simulink model "assignment_1"  (R2022a)
settings: Solver=FixedStepAuto  StartTime=0.0  StopTime=inf  FixedStep=1e-3  RelTol=1e-3  EnableMultiTasking=on
undefined symbols (not defined in the file): D0, D1, D10, D11, D12, D13, D2, D3, D4, D5, D6, D7, D8, D9, PTA0, PTA1, PTA2, PTB23, PTB9, PTC16, PTC17, PTC2, PTC3, PTC4, PTD0, PTD1, PTD2, PTD3
libraries: frdmk64flib x16
settings Model: ExtModeTrigDuration=5  Creator=Xu Yue  LastModifiedBy=Xu Yue
settings OptimizationCC: EnhancedBackFolding=on  PassReuseOutputArgsAs=Individual arguments  ZeroExternalMemoryAtStartup=off  ZeroInternalMemoryAtStartup=off  MaxStackSize=64  OptimizeBlockOrder=speed  DifferentSizesBufferReuse=on  OptimizationCustomize=off  EfficientTunableParamExpr=on
settings DebuggingCC: ParameterTunabilityLossMsg=error
settings HardwareCC: ProdBitPerPointer=32  ProdBitPerSizeT=32  ProdBitPerPtrDiffT=32  ProdLargestAtomicInteger=Long  ProdLargestAtomicFloat=Double  ProdWordSize=32  ProdHWDeviceType=ARM Compatible->ARM Cortex
settings SFSimCC: MATLABDynamicMemAlloc=off
settings RTWCC: SystemTargetFile=ert.tlc  HardwareBoard=NXP FRDM-K64F  TLCOptions="-aInlineSetEventsForThisBaseRateFcn=TLC_FALSE -aSuppressMultiTaskScheduler=TLC_FALSE  -aRateBasedStepFcn=0"  TemplateMakefile=ert_default_tmf  Toolchain=GNU Tools for ARM Embedded Processors
settings CodeAppCC: ForceParamTrailComments=on  IgnoreCustomStorageClasses=off  OperatorAnnotations=on  SimulinkDataObjDesc=on  SFDataObjDesc=on  InsertBlockDesc=on
settings ERTTargetCC: SupportContinuousTime=on  ExtModeTransport=4  ExtModeMexFile=sendToCommService

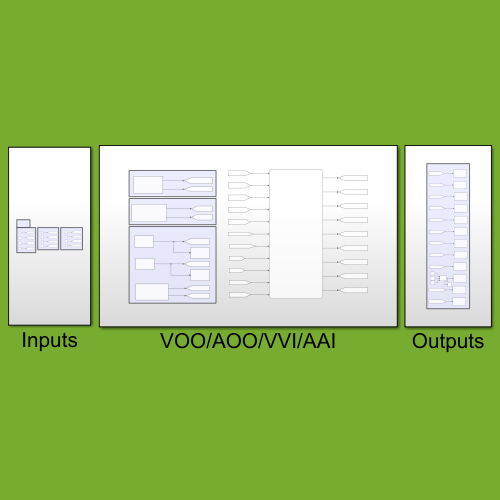
[thumbnail: Simulink's stored preview of the top-level diagram]
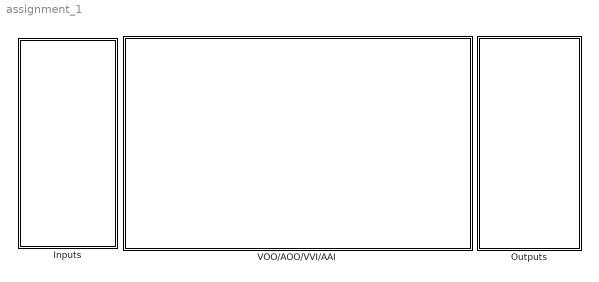
== system assignment_1 ==
  Inputs : Subsystem
  Outputs : Subsystem
  VOO/AOO/VVI/AAI : Subsystem

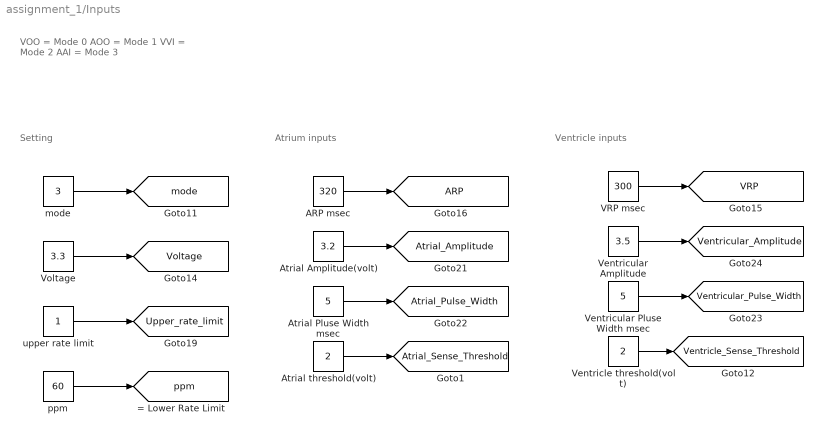
== system assignment_1/Inputs ==
  note: VOO = Mode 0
      | AOO = Mode 1
      | VVI = Mode 2
      | AAI = Mode 3
  note: Atrium inputs
  note: Setting
  note: Ventricle inputs
  ARP msec : Constant  Value=320
  Atrial Amplitude(volt) : Constant  Value=3.2
  Atrial Pluse Width msec : Constant  Value=5
  Atrial threshold(volt) : Constant  Value=2
  VRP msec : Constant  Value=300
  Ventricle threshold(volt) : Constant  Value=2
  Ventricular Amplitude : Constant  Value=3.5
  Ventricular Pluse Width msec : Constant  Value=5
  Voltage : Constant  Value=3.3
  mode : Constant  Value=3
  ppm : Constant  Value=60
  upper rate limit : Constant
  tag scope: ARP=global, Atrial_Amplitude=global, Atrial_Pulse_Width=global, Atrial_Sense_Threshold=global, Upper_rate_limit=global, VRP=global, Ventricle_Sense_Threshold=global, Ventricular_Amplitude=global, Ventricular_Pulse_Width=global, Voltage=global, mode=global, ppm=global
  wires:
  Ventricular Pluse Width msec/1 -> [Ventricular_Pulse_Width]
  Voltage/1 -> [Voltage]
  ppm/1 -> [ppm]
  mode/1 -> [mode]
  Ventricular Amplitude/1 -> [Ventricular_Amplitude]
  VRP msec/1 -> [VRP]
  upper rate limit/1 -> [Upper_rate_limit]
  Atrial Pluse Width msec/1 -> [Atrial_Pulse_Width]
  ARP msec/1 -> [ARP]
  Atrial Amplitude(volt)/1 -> [Atrial_Amplitude]
  Atrial threshold(volt)/1 -> [Atrial_Sense_Threshold]
  Ventricle threshold(volt)/1 -> [Ventricle_Sense_Threshold]

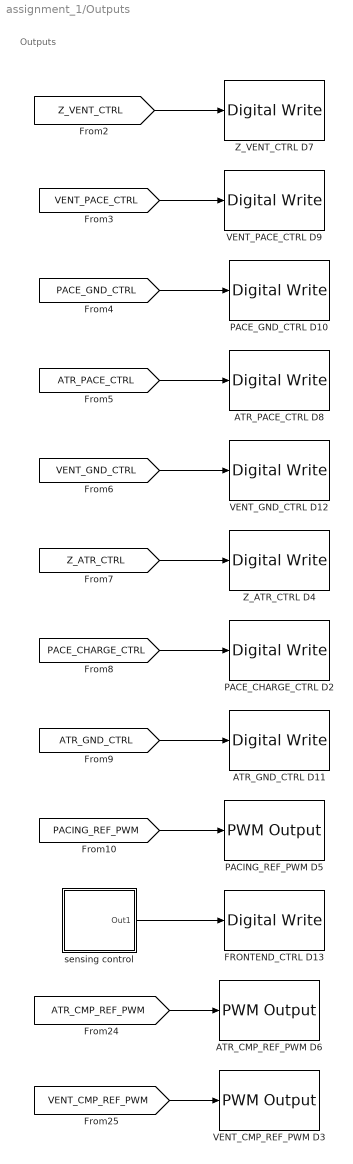
== system assignment_1/Outputs ==
  note: Outputs
  ATR_CMP_REF_PWM D6 : frdmk64flib/PWM Output  Whichpin=PTC2 (D6)  InitialFrequency=2000  InitialDutyCycle=0
  ATR_GND_CTRL D11 : frdmk64flib/Digital Write  Whichpin=PTD2 (D11)
  ATR_PACE_CTRL D8 : frdmk64flib/Digital Write  Whichpin=PTA0 (D8)
  FRONTEND_CTRL D13 : frdmk64flib/Digital Write  Whichpin=PTD1 (D13)
  PACE_CHARGE_CTRL D2 : frdmk64flib/Digital Write  Whichpin=PTB9 (D2)
  PACE_GND_CTRL D10 : frdmk64flib/Digital Write  Whichpin=PTD0 (D10)
  PACING_REF_PWM D5 : frdmk64flib/PWM Output  Whichpin=PTA2 (D5)  InitialFrequency=2000  InitialDutyCycle=0
  VENT_CMP_REF_PWM D3 : frdmk64flib/PWM Output  Whichpin=PTA1 (D3)  InitialFrequency=2000  InitialDutyCycle=0
  VENT_GND_CTRL D12 : frdmk64flib/Digital Write  Whichpin=PTD3 (D12)
  "VENT_PACE_CTRL D9  " : frdmk64flib/Digital Write  Whichpin=PTC4 (D9)
  Z_ATR_CTRL D4 : frdmk64flib/Digital Write  Whichpin=PTB23 (D4)
  Z_VENT_CTRL D7 : frdmk64flib/Digital Write  Whichpin=PTC3 (D7)
  sensing control : Subsystem
  wires:
  [VENT_GND_CTRL] -> VENT_GND_CTRL D12/1
  [ATR_PACE_CTRL] -> ATR_PACE_CTRL D8/1
  [PACE_CHARGE_CTRL] -> PACE_CHARGE_CTRL D2/1
  [VENT_PACE_CTRL] -> "VENT_PACE_CTRL D9  "/1
  [Z_VENT_CTRL] -> Z_VENT_CTRL D7/1
  [PACE_GND_CTRL] -> PACE_GND_CTRL D10/1
  [Z_ATR_CTRL] -> Z_ATR_CTRL D4/1
  [PACING_REF_PWM] -> PACING_REF_PWM D5/1
  [ATR_CMP_REF_PWM] -> ATR_CMP_REF_PWM D6/1
  [VENT_CMP_REF_PWM] -> VENT_CMP_REF_PWM D3/1
  [ATR_GND_CTRL] -> ATR_GND_CTRL D11/1
  sensing control/1(Out1) -> FRONTEND_CTRL D13/1

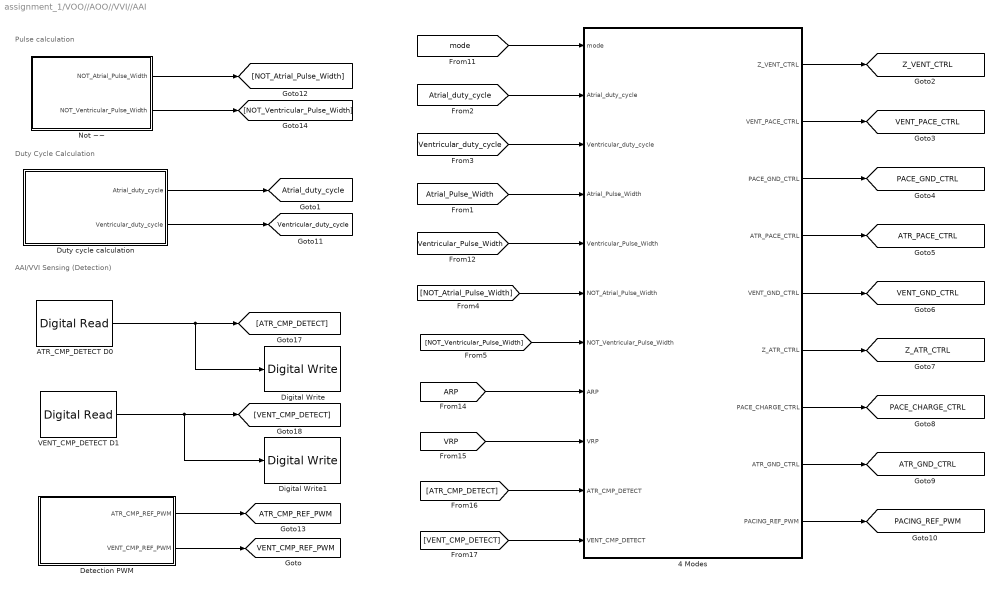
== system assignment_1/VOO//AOO//VVI//AAI ==
  note: Duty Cycle Calculation
  note: Pulse calculation
  note: AAI/VVI Sensing (Detection)
  4 Modes : Stateflow chart  TreatAsAtomicUnit=on
  ATR_CMP_DETECT D0 : frdmk64flib/Digital Read  Whichpin=PTC16 (D0)  SampleTime=-1
  Detection PWM : Subsystem
  Digital Write : frdmk64flib/Digital Write  Whichpin=RED_LED
  Digital Write1 : frdmk64flib/Digital Write  Whichpin=BLUE_LED
  Duty cycle calculation : Subsystem
  Not ~~ : Subsystem
  VENT_CMP_DETECT D1 : frdmk64flib/Digital Read  Whichpin=PTC17 (D1)  SampleTime=-1
  tag scope: ATR_CMP_REF_PWM=global, ATR_GND_CTRL=global, ATR_PACE_CTRL=global, Atrial_duty_cycle=global, PACE_CHARGE_CTRL=global, PACE_GND_CTRL=global, PACING_REF_PWM=global, VENT_CMP_REF_PWM=global, VENT_GND_CTRL=global, VENT_PACE_CTRL=global, Ventricular_duty_cycle=global, Z_ATR_CTRL=global, Z_VENT_CTRL=global
  wires:
  4 Modes/5(VENT_GND_CTRL) -> [VENT_GND_CTRL]
  4 Modes/1(Z_VENT_CTRL) -> [Z_VENT_CTRL]
  4 Modes/8(ATR_GND_CTRL) -> [ATR_GND_CTRL]
  Detection PWM/1(ATR_CMP_REF_PWM) -> [ATR_CMP_REF_PWM]
  [mode] -> 4 Modes/1(mode)
  4 Modes/6(Z_ATR_CTRL) -> [Z_ATR_CTRL]
  4 Modes/3(PACE_GND_CTRL) -> [PACE_GND_CTRL]
  4 Modes/9(PACING_REF_PWM) -> [PACING_REF_PWM]
  [ATR_CMP_DETECT] -> 4 Modes/10(ATR_CMP_DETECT)
  4 Modes/2(VENT_PACE_CTRL) -> [VENT_PACE_CTRL]
  ATR_CMP_DETECT D0/1 -> Digital Write/1, [ATR_CMP_DETECT]
  [VENT_CMP_DETECT] -> 4 Modes/11(VENT_CMP_DETECT)
  [Atrial_Pulse_Width] -> 4 Modes/4(Atrial_Pulse_Width)
  [ARP] -> 4 Modes/8(ARP)
  [Ventricular_Pulse_Width] -> 4 Modes/5(Ventricular_Pulse_Width)
  4 Modes/4(ATR_PACE_CTRL) -> [ATR_PACE_CTRL]
  [VRP] -> 4 Modes/9(VRP)
  4 Modes/7(PACE_CHARGE_CTRL) -> [PACE_CHARGE_CTRL]
  Detection PWM/2(VENT_CMP_REF_PWM) -> [VENT_CMP_REF_PWM]
  Duty cycle calculation/1(Atrial_duty_cycle) -> [Atrial_duty_cycle]
  Duty cycle calculation/2(Ventricular_duty_cycle) -> [Ventricular_duty_cycle]
  [Atrial_duty_cycle] -> 4 Modes/2(Atrial_duty_cycle)
  [Ventricular_duty_cycle] -> 4 Modes/3(Ventricular_duty_cycle)
  Not ~~/1(NOT_Atrial_Pulse_Width) -> [NOT_Atrial_Pulse_Width]
  Not ~~/2(NOT_Ventricular_Pulse_Width) -> [NOT_Ventricular_Pulse_Width]
  [NOT_Atrial_Pulse_Width] -> 4 Modes/6(NOT_Atrial_Pulse_Width)
  [NOT_Ventricular_Pulse_Width] -> 4 Modes/7(NOT_Ventricular_Pulse_Width)
  VENT_CMP_DETECT D1/1 -> Digital Write1/1, [VENT_CMP_DETECT]

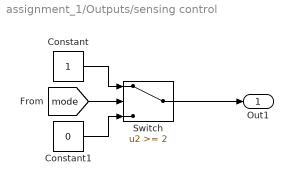
== system assignment_1/Outputs/sensing control ==
  Constant : Constant
  Constant1 : Constant  Value=0
  Switch : Switch  Threshold=2  SaturateOnIntegerOverflow=off  InputSameDT=off
  Out1 : Outport
  wires:
  Constant/1 -> Switch/1
  Constant1/1 -> Switch/3
  [mode] -> Switch/2
  Switch/1 -> Out1/1

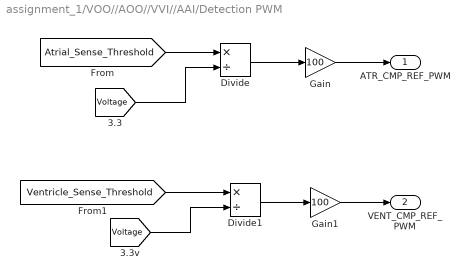
== system assignment_1/VOO//AOO//VVI//AAI/Detection PWM ==
  Divide : Product  Inputs=*/  RndMeth=Zero  SaturateOnIntegerOverflow=on
  Divide1 : Product  Inputs=*/  RndMeth=Zero  SaturateOnIntegerOverflow=on
  Gain : Gain  Gain=100
  Gain1 : Gain  Gain=100
  ATR_CMP_REF_PWM : Outport
  VENT_CMP_REF_PWM : Outport  Port=2
  wires:
  Divide/1 -> Gain/1
  Gain/1 -> ATR_CMP_REF_PWM/1
  [Voltage] -> Divide1/2
  Divide1/1 -> Gain1/1
  Gain1/1 -> VENT_CMP_REF_PWM/1
  [Voltage] -> Divide/2
  [Atrial_Sense_Threshold] -> Divide/1
  [Ventricle_Sense_Threshold] -> Divide1/1

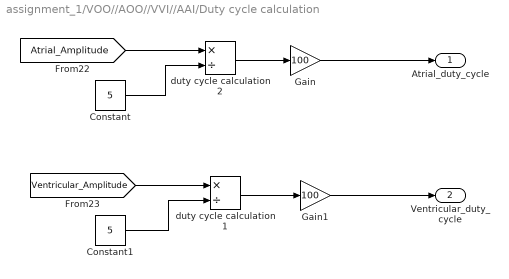
== system assignment_1/VOO//AOO//VVI//AAI/Duty cycle calculation ==
  Constant : Constant  Value=5
  Constant1 : Constant  Value=5
  Gain : Gain  Gain=100
  Gain1 : Gain  Gain=100
  duty cycle calculation1 : Product  Inputs=*/  RndMeth=Zero  SaturateOnIntegerOverflow=on
  duty cycle calculation2 : Product  Inputs=*/  RndMeth=Zero  SaturateOnIntegerOverflow=on
  Atrial_duty_cycle : Outport
  Ventricular_duty_cycle : Outport  Port=2
  wires:
  Gain/1 -> Atrial_duty_cycle/1
  Gain1/1 -> Ventricular_duty_cycle/1
  duty cycle calculation1/1 -> Gain1/1
  duty cycle calculation2/1 -> Gain/1
  Constant1/1 -> duty cycle calculation1/2
  Constant/1 -> duty cycle calculation2/2
  [Ventricular_Amplitude] -> duty cycle calculation1/1
  [Atrial_Amplitude] -> duty cycle calculation2/1

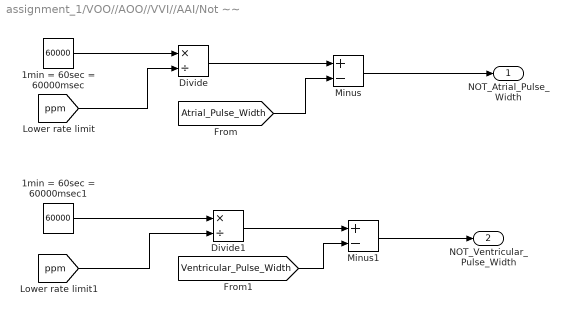
== system assignment_1/VOO//AOO//VVI//AAI/Not ~~ ==
  1min = 60sec = 60000msec : Constant  Value=60000
  1min = 60sec = 60000msec1 : Constant  Value=60000
  Divide : Product  Inputs=*/
  Divide1 : Product  Inputs=*/
  Minus : Sum  Inputs=+-
  Minus1 : Sum  Inputs=+-
  NOT_Atrial_Pulse_Width : Outport
  NOT_Ventricular_Pulse_Width : Outport  Port=2
  wires:
  1min = 60sec = 60000msec/1 -> Divide/1
  Divide/1 -> Minus/1
  Minus/1 -> NOT_Atrial_Pulse_Width/1
  1min = 60sec = 60000msec1/1 -> Divide1/1
  Divide1/1 -> Minus1/1
  Minus1/1 -> NOT_Ventricular_Pulse_Width/1
  [ppm] -> Divide/2
  [ppm] -> Divide1/2
  [Atrial_Pulse_Width] -> Minus/2
  [Ventricular_Pulse_Width] -> Minus1/2

== stateflow chart assignment_1/VOO//AOO//VVI//AAI/4 Modes ==
  state VOO
    state VOO [group]
      state Charging
        entry:
        %Charging C22
        ATR_PACE_CTRL = LOW
        VENT_PACE_CTRL = LOW
        PACING_REF_PWM = Ventricular_duty_cycle
        PACE_CHARGE_CTRL = HIGH
        %Discharging Blocking Cap C21
        PACE_GND_CTRL = HIGH
        VENT_PACE_CTRL = LOW
        Z_ATR_CTRL = LOW
        Z_VENT_CTRL = LOW
        ATR_PACE_CTRL = LOW
        ATR_GND_CTRL = LOW
        VENT_GND_CTRL = HIGH
      state Pacing
        entry:
        %Discharge C22 (Charge C21)
        PACE_CHARGE_CTRL = LOW
        PACE_GND_CTRL = HIGH
        ATR_PACE_CTRL = LOW
        ATR_GND_CTRL = LOW
        Z_ATR_CTRL = LOW
        Z_VENT_CTRL = LOW
        VENT_GND_CTRL = LOW
        VENT_PACE_CTRL = HIGH
      VOO.VOO.Charging -> VOO.VOO.Pacing [order 1] : [after(NOT_Ventricular_Pulse_Width,msec)]
      VOO.VOO.Pacing -> VOO.VOO.Charging : [after(Ventricular_Pulse_Width,msec)]
  state Start
    % mode 0 = VOO
    % mode 1 = AOO
    % mode 2 = VVI
    % mode 3 = AAI
  state AOO
    state AOO [group]
      state Charging
        entry:
        %Charging C22
        ATR_PACE_CTRL = LOW
        VENT_PACE_CTRL = LOW
        PACING_REF_PWM = Atrial_duty_cycle
        PACE_CHARGE_CTRL = HIGH
        %Discharging Blocking Cap C21
        PACE_GND_CTRL = HIGH
        VENT_PACE_CTRL = LOW
        Z_ATR_CTRL = LOW
        Z_VENT_CTRL = LOW
        ATR_PACE_CTRL = LOW
        ATR_GND_CTRL = HIGH
        VENT_GND_CTRL = LOW
      state Pacing
        entry:
        %Discharge C22 (Charge C21)
        PACE_CHARGE_CTRL = LOW
        PACE_GND_CTRL = HIGH
        ATR_PACE_CTRL = HIGH
        ATR_GND_CTRL = LOW
        Z_ATR_CTRL = LOW
        Z_VENT_CTRL = LOW
        VENT_GND_CTRL = LOW
        VENT_PACE_CTRL = LOW
      AOO.AOO.Charging -> AOO.AOO.Pacing [order 1] : after(NOT_Atrial_Pulse_Width,msec)
      AOO.AOO.Pacing -> AOO.AOO.Charging : after(Atrial_Pulse_Width,msec)
  state VVI
    state VVI [group]
      state Pacing
        entry:
        %Discharge C22 (Charge C21)
        PACE_CHARGE_CTRL = LOW
        PACE_GND_CTRL = HIGH
        ATR_PACE_CTRL = LOW
        ATR_GND_CTRL = LOW
        Z_ATR_CTRL = LOW
        Z_VENT_CTRL = LOW
        VENT_GND_CTRL = LOW
        VENT_PACE_CTRL = HIGH
      state Alert_Period
        %If nature pace occur
        %go back to VRP_Period
      state Charging1
        entry:
        %Charging C22
        ATR_PACE_CTRL = LOW
        VENT_PACE_CTRL = LOW
        PACING_REF_PWM = Ventricular_duty_cycle
        PACE_CHARGE_CTRL = HIGH
        %Discharging Blocking Cap C21
        PACE_GND_CTRL = HIGH
        VENT_PACE_CTRL = LOW
        Z_ATR_CTRL = LOW
        Z_VENT_CTRL = LOW
        ATR_PACE_CTRL = LOW
        ATR_GND_CTRL = LOW
        VENT_GND_CTRL = HIGH
      state VRP_Period
        %refractory period
      VVI.VVI.Alert_Period -> VRP_Period [order 1] : [VENT_CMP_DETECT ==  true]
      VVI.VVI.Alert_Period -> VVI.VVI.Pacing [order 2] : after(NOT_Ventricular_Pulse_Width - VRP,msec)
      VRP_Period -> VVI.VVI.Alert_Period : after(VRP, msec)
      Charging1 -> VRP_Period [order 2]
      VVI.VVI.Pacing -> Charging1 : after(Ventricular_Pulse_Width,msec)
  state AAI
    state AAI [group]
      state Charging
        entry:
        %Charging C22
        ATR_PACE_CTRL = LOW
        VENT_PACE_CTRL = LOW
        PACING_REF_PWM = Atrial_duty_cycle
        PACE_CHARGE_CTRL = HIGH
        %Discharging Blocking Cap C21
        PACE_GND_CTRL = HIGH
        VENT_PACE_CTRL = LOW
        Z_ATR_CTRL = LOW
        Z_VENT_CTRL = LOW
        ATR_PACE_CTRL = LOW
        ATR_GND_CTRL = HIGH
        VENT_GND_CTRL = LOW
      state Alert_Period
        %If nature pace occur
        %reset ARP_Period
      state Pacing
        entry:
        %Discharge C22 (Charge C21)
        PACE_CHARGE_CTRL = LOW
        PACE_GND_CTRL = HIGH
        ATR_PACE_CTRL = HIGH
        ATR_GND_CTRL = LOW
        Z_ATR_CTRL = LOW
        Z_VENT_CTRL = LOW
        VENT_GND_CTRL = LOW
        VENT_PACE_CTRL = LOW
      state ARP_Period
        %refractory period
      AAI.AAI.Alert_Period -> ARP_Period [order 1] : [ATR_CMP_DETECT == true]
      AAI.AAI.Alert_Period -> AAI.AAI.Pacing [order 2] : after(NOT_Atrial_Pulse_Width - ARP, msec)
      ARP_Period -> AAI.AAI.Alert_Period : after(ARP, msec)
      AAI.AAI.Charging -> ARP_Period [order 2]
      AAI.AAI.Pacing -> AAI.AAI.Charging : after(Atrial_Pulse_Width, msec)
  (default) -> Start
  AOO.AOO.Charging -> Start [order 2] : [mode ~= 1]
  Charging1 -> Start [order 1] : [mode ~= 2]
  AAI.AAI.Charging -> Start [order 1] : [mode ~= 3]
  VOO.VOO.Charging -> Start [order 2] : [mode ~= 0]
  Start -> VOO.VOO.Charging [order 2] : [mode == 0]
  Start -> AOO.AOO.Charging [order 3] : [mode == 1]
  Start -> Charging1 [order 1] : [mode == 2]
  Start -> AAI.AAI.Charging [order 4] : [mode == 3]
  data: mode input; Z_VENT_CTRL output; VENT_PACE_CTRL output; PACE_GND_CTRL output; ATR_PACE_CTRL output; VENT_GND_CTRL output; Z_ATR_CTRL output; PACE_CHARGE_CTRL output; ATR_GND_CTRL output; PACING_REF_PWM output; LOW constant boolean =0; HIGH constant boolean =1; Atrial_duty_cycle input; Ventricular_duty_cycle input; Atrial_Pulse_Width input; Ventricular_Pulse_Width input; NOT_Atrial_Pulse_Width input; NOT_Ventricular_Pulse_Width input; ARP input; VRP input; ATR_CMP_DETECT input; VENT_CMP_DETECT input
